simulink model "test"  (R2021b)
settings: Solver=VariableStepAuto  StartTime=0.0  StopTime=600  RelTol=1e-3
values from neighbouring files (symbols this model uses):
  floor_height = 3    [load_data.m]
  g = 9.806    [load_data.m]
  Ts = 1e-3    (= 0.001)    [load_data.m]
libraries: LiftMotionControlLibrary x6, LumpedParameterLiftModels x2, simulink_extras x1
settings Model: Creator=manue  LastModifiedBy=manue
settings ConfigComp: PLC_TargetIDE=generic  PLC_MultiTBSigbuilderTimeRange=off  PLC_InlineEnumCastFunction=off

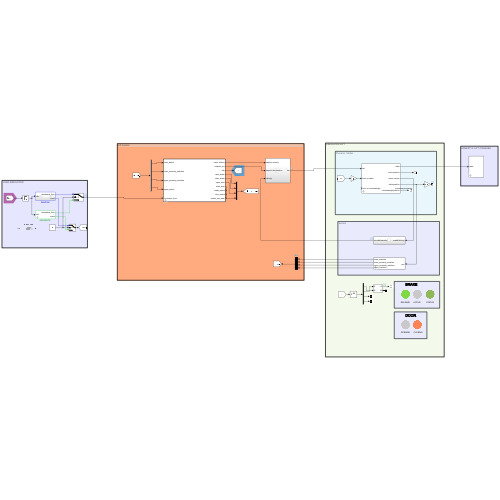
[thumbnail: Simulink's stored preview of the top-level diagram]
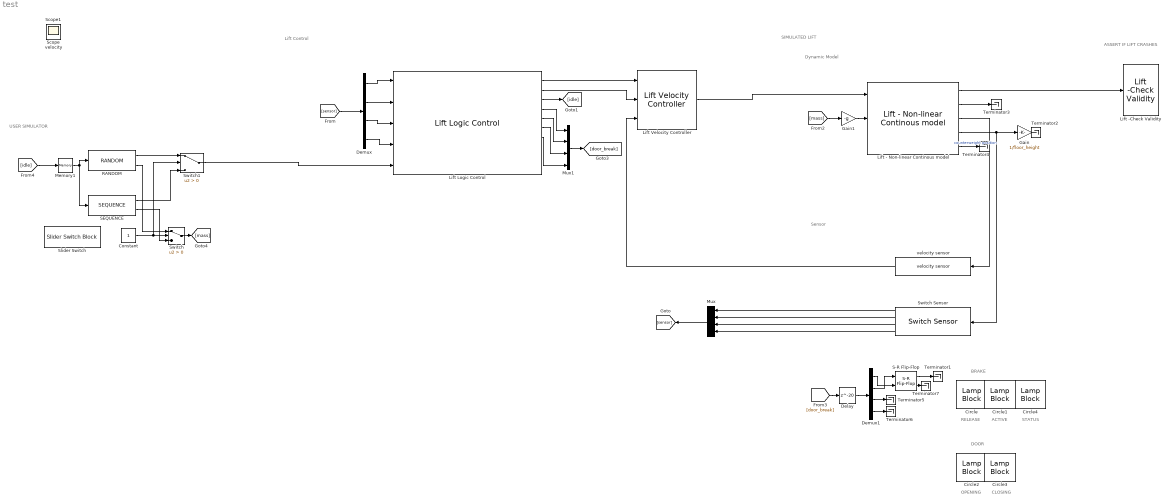
== system test ==
  note: RELEASE
  note: BRAKE
  note: ASSERT IF LIFT CRASHES
  note: SIMULATED LIFT
  note: Sensor
  note: Dynamic Model
  note: Lift Control
  note: ACTIVE
  note: DOOR
  note: OPENING
  note: CLOSING
  note: STATUS
  note: USER SIMULATOR
  Circle{,1..4} (5 alike) : LampBlock  LabelPosition=Hide  Icon=Circle
  Constant : Constant
  Delay : Delay  DelayLength=20  SampleTime=Ts
  Demux : Demux
  Demux1 : Demux
  Gain : Gain  Gain=1/floor_height
  Gain1 : Gain  Gain=-g
  Lift - Non-linear Continous model : LumpedParameterLiftModels/Lift - Non-linear Continous model  Jp=Jp  Jm=Jm  Mc=Mc  Mw=Mw  LinearStiffness=LinearStiffness  LinearDamping=LinearDamping  Rp=Rp  mu=mu  BuildingHeight=BuildingHeight  MotorViscousFriction=MotorViscousFriction  g=g  gearbox=gearbox  min_length=min_length  x9_init=0
  Lift -Check Validity : LumpedParameterLiftModels/Lift -Check Validity  BuildingHeight=BuildingHeight  min_length=3
  Lift Logic Control : LiftMotionControlLibrary/Lift Logic Control  num_floors=num_floors  Ts=Ts  gearbox=gearbox  Rp=Rp  waiting_time_open_door=waiting_time_open_door  waiting_time_close_door=waiting_time_close_door  waiting_time_open_brake=waiting_time_open_brake  waiting_time_close_brake_copy=waiting_time_close_brake  waiting_time_steady_state=waiting_time_steady_state  HighSpeed=HighSpeed  LowSpeed=LowSpeed  PercentAccFactor=PercentAccFactor  AccelInitialJerk=AccelInitialJerk  Acceleration=Acceleration  AccelEndJerk=AccelEndJerk  DecelInitialJerk=DecelInitialJerk  Deceleration=Deceleration  DecelEndJerk=DecelEndJerk  StopDeceleration=StopDeceleration
  Lift Velocity Controller : LiftMotionControlLibrary/Lift Velocity Controller  SystemSampleTime=-1  VariantActivationTime=update diagram  Latency=0  AutoFrameSizeCalculation=off
  Memory1 : Memory
  Mux : Mux
  Mux1 : Mux
  "RANDOM " : LiftMotionControlLibrary/RANDOM  SystemSampleTime=-1  VariantActivationTime=update diagram  Latency=0  AutoFrameSizeCalculation=off
  S-R Flip-Flop : simulink_extras/Flip Flops/S-R Flip-Flop  initial_condition=1
  "SEQUENCE " : LiftMotionControlLibrary/SEQUENCE  sequence=[10]
  Slider Switch : SliderSwitchBlock
      settings: Values={{'SEQUENCE', 'RANDOM'}, [0 1]}
  Switch : Switch  Criteria=u2 > Threshold
  Switch Sensor : LiftMotionControlLibrary/Switch Sensor  lower_proximity_sensor_positions=lower_proximity_sensor_positions  upper_proximity_sensor_positions=upper_proximity_sensor_positions  lower_floor_sensor_positions=lower_floor_sensor_positions  upper_floor_sensor_positions=upper_floor_sensor_positions  num_floors=num_floors  sensor_height=sensor_height
  Switch1 : Switch  Criteria=u2 > Threshold
  Terminator{1..7} (7 alike) : Terminator
  velocity sensor : LiftMotionControlLibrary/velocity sensor  SystemSampleTime=-1  VariantActivationTime=update diagram  Latency=0  AutoFrameSizeCalculation=off
  Scope : Scope
  Scope1 : Scope
  velocity : Scope
  wires:
  Lift - Non-linear Continous model/4 -> Gain/1, Switch Sensor/1
  Switch Sensor/1 -> Mux/1
  Switch Sensor/2 -> Mux/2
  Switch Sensor/3 -> Mux/3
  Demux/3 -> Lift Logic Control/3
  Demux/2 -> Lift Logic Control/2
  Demux/1 -> Lift Logic Control/1
  Mux/1 -> [sensor]
  [sensor] -> Demux/1
  Lift Logic Control/1 -> Lift Velocity Controller/1
  velocity sensor/1 -> Lift Velocity Controller/3
  Lift Velocity Controller/1 -> Lift - Non-linear Continous model/1
  Lift Logic Control/2 -> Lift Velocity Controller/2
  Lift Logic Control/3 -> [idle]
  [mass] -> Gain1/1
  Lift - Non-linear Continous model/3 -> velocity sensor/1
  Gain/1 -> Terminator2/1
  Lift - Non-linear Continous model/1 -> Lift -Check Validity/1
  Lift - Non-linear Continous model/2 -> Terminator3/1
  Lift - Non-linear Continous model/5 -> Terminator4/1  "counterweight position"
  Gain1/1 -> Lift - Non-linear Continous model/2
  Lift Logic Control/5 -> Mux1/2
  Lift Logic Control/4 -> Mux1/1
  Lift Logic Control/6 -> Mux1/3
  Lift Logic Control/7 -> Mux1/4
  Mux1/1 -> [door_break]
  [door_break] -> Delay/1
  Demux1/3 -> Terminator5/1
  Demux1/4 -> Terminator6/1
  Demux1/1 -> S-R Flip-Flop/2
  Demux1/2 -> S-R Flip-Flop/1
  S-R Flip-Flop/1 -> Terminator1/1
  S-R Flip-Flop/2 -> Terminator7/1
  Constant/1 -> Switch1/2, Switch/2
  "SEQUENCE "/1 -> Switch1/3
  "RANDOM "/1 -> Switch1/1
  Switch/1 -> [mass]
  Memory1/1 -> "SEQUENCE "/1, "RANDOM "/1
  "SEQUENCE "/2 -> Switch/3
  [idle] -> Memory1/1
  "RANDOM "/2 -> Switch/1
  Switch1/1 -> Lift Logic Control/5
  Delay/1 -> Demux1/1
  Switch Sensor/4 -> Mux/4
  Demux/4 -> Lift Logic Control/4
